simulink model "sl_jspace"  (R2015a)
settings: Solver=ode45  StartTime=0.0  StopTime=5  RelTol=1e-3
InitFcn:
  | if ~exist('p560')
  |   mdl_puma560
  | end
libraries: roblocks x4, simulink x1
settings Model: ExtModeTrigMode=oneshot  ExtModeArmWhenConnect=off  ExtModeAutoUpdateStatusClock=off  Creator=pic  LastModifiedBy=corkep
settings DataIOCC: LimitDataPoints=off  SignalLoggingSaveFormat=ModelDataLogs  SignalLoggingName=sigsOut
settings OptimizationCC: BlockReduction=off  BooleanDataType=off  ExpressionDepthLimit=2147483647
settings DebuggingCC: SaveWithParameterizedLinksMsg=none  UnderspecifiedInitializationDetection=Classic  MergeDetectMultiDrivingBlocksExec=none  SignalResolutionControl=TryResolveAllWithWarning  MultiTaskDSMMsg=warning  MultiTaskCondExecSysMsg=none  StateNameClashWarn=warning
settings HardwareCC: TargetUnknown=on
settings GRTTargetCC: CombineOutputUpdateFcns=off  GRTInterface=on

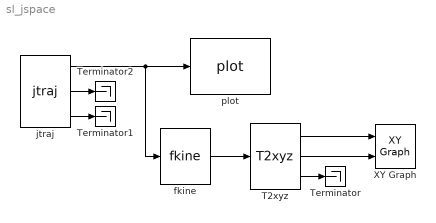
== system sl_jspace ==
  T2xyz : roblocks/Toolbox/T2xyz
  Terminator : Terminator
  Terminator1 : Terminator
  Terminator2 : Terminator
  XY Graph : simulink/Sinks/XY Graph  xmin=-1  xmax=1  ymin=-1  ymax=1  st=-1
  fkine : roblocks/Arm/fkine  robot=p560
  jtraj : roblocks/Toolbox/jtraj  q0=[0 0 0 0 0 0]  qf=[pi/4 pi/2 -pi/2 0 0 0]  tmax=5  ts=0.02
  plot : roblocks/Arm/plot  robot=p560  fps=25  holdplot=on
  wires:
  jtraj/1 -> plot/1, fkine/1
  fkine/1 -> T2xyz/1
  T2xyz/1 -> XY Graph/1
  T2xyz/2 -> XY Graph/2
  jtraj/2 -> Terminator2/1
  jtraj/3 -> Terminator1/1
  T2xyz/3 -> Terminator/1
